simulink model "PLANTA_CONTROL_OBS"  (R2024b)
settings: Solver=FixedStepAuto  StartTime=0.0  StopTime=inf  FixedStep=0.001  MaxStep=0.0005  RelTol=1e-4
InitFcn:
  | load('ml_breakpoints.mat')
  | load('l_breakpoints.mat')
  | load('at_breakpoints.mat')
  | load('Kp_table.mat')
  | load('Kd_table.mat')
undefined symbols (not defined in the file): A_hm, A_tm, at_breakpoints, at_max, b_ha, B_hm, b_ta, B_tm, bcx, bcy, bhd, bhEb, bhm, bt, btd, btm, btw, bwu, C_hm, C_tm, D_hm, D_tm, DiscIntNeverNeededParam, dl_h_ini, dx_l_ini, dx_t_ini, dx_td_ini, dxt_max, dy_l_ini, F01_a_t_max, F01_Ts1, F02_a_h_max, F02_Ts1, F03_a_h_max, F03_a_t_max, F03_dxt_max, F03_Ts1, Fhw_min, g, Hc, ih, it, Jhd_hEb, Jhm_hb, Jtd, Jtm_tb, K_hsa, K_hsia, K_tsa, K_tsia, Kcy, Kd_table, Ke_tita, Ke_w, kp_pos, Kp_table, kp_w, Ktw, kwu, l_breakpoints ... (+26)
libraries: simulink x7, spsEdgeDetectorLib x5, simulink_extras x2, dspsigops x2, vrlib x1, dspstat3 x1
(part 4 of 4)

== stateflow chart PLANTA_CONTROL_OBS/Nivel 1 - Control Supervisor ==
  state PERFIL_DE_OBSTACULOS [parallel]
    entry:
    num_index = floor(80/Wc);
    Y_perfil = zeros(1,num_index,'double');
    during:
    %xtd = theta_mt*pulsos_x_rev*dist_x_pulso*(1/100);
    xtd_lidar = (xtd+30)+3;
    index = floor(xtd_lidar/Wc);
    Y_c0_read = yc0_xt;
    if index>0 && index<=32
    Y_perfil(index) = Y_c0_read;
    end
    settings: executionOrder=2
  state OFF [parallel]
    settings: executionOrder=1
    state EMERGENCIA
      entry:
      %Cuando el control supervisor entra en esta de emergencia, cede
      %el control al Nivel 0 hasta retomar el estado normal
      dxt_ref=0;
      dlh_ref=0;
      ddxt_ref=0;
    state ON
      entry:
      dxt_ref_ant = 0;
      dlh_ref_ant = 0;
      dxt_ref = 0;
      dlh_ref = 0;
      ddxt_ref = 0;
      state DETECCION_ESTADOS [parallel]
        settings: executionOrder=1
        state TWISTLOCKS [parallel]
          settings: executionOrder=1
          state VERIFICAR
          state ACT_TLK
            entry:
            TLK=1;
            c=-ceil((xtd+30)/Wc);
            during:
            y_real=45-(lh+Hc);
          state DES_TLK
            entry:
            TLK=0;
            c=ceil((xtd+30)/Wc);
            during:
            y_real=45-lh;
          (default) -> VERIFICAR
          VERIFICAR -> ACT_TLK [order 2] : [TLK_act==1]
          VERIFICAR -> DES_TLK [order 1] : [TLK_act==0]
          ACT_TLK -> DES_TLK : [TLK_act==0 && op_mode==1 && cable_tenso==0]
          DES_TLK -> ACT_TLK : [TLK_act==1 && op_mode==1 && cable_tenso==0]
        state FRENOS [parallel]
          settings: executionOrder=2
          state FRENO_IZAJE [parallel]
            settings: executionOrder=1
            state FRENO_IZAJE_OFF
              entry:
              BRK_h=1;
              parar_izaje=0;
            state FRENO_IZAJE_ON
              entry:
              BRK_h=0;
              parar_izaje=1;
            (default) -> FRENO_IZAJE_ON
            FRENO_IZAJE_OFF -> FRENO_IZAJE_ON : [(abs(whm)<=whm_min && (abs(whm) < abs(whm_ant)-(whm_min*0.01)))]
            FRENO_IZAJE_ON -> FRENO_IZAJE_OFF : [abs(Thm_disp) && (abs(dlh_ref)>0.1 || dlh_ref_man~=0) && after(0.2,sec)]
          state FRENO_CARRO [parallel]
            settings: executionOrder=2
            state FRENO_CARRO_OFF
              entry:
              BRK_t=1;
              parar_carro=0;
            state FRENO_CARRO_ON
              entry:
              BRK_t=0;
              parar_carro=1;
            (default) -> FRENO_CARRO_ON
            FRENO_CARRO_OFF -> FRENO_CARRO_ON : [(abs(wtm)<=wtm_min && (abs(wtm)<abs(wtm_ant)-wtm_min*0.01))]
            FRENO_CARRO_ON -> FRENO_CARRO_OFF : [abs(Ttm_disp) && (abs(dxt_ref)>0.1 || dxt_ref_man~=0) && after(0.2,sec)]
        state FINALES [parallel]
          settings: executionOrder=3
          state FIN_CARRERA_CARRO [parallel]
            settings: executionOrder=1
            state PARAR_CARRO
              entry:
              op_mode=1;
              parar_carro=1;
            state MOVER_CARRO
              entry:
              parar_carro=0;
            (default) -> MOVER_CARRO
            OFF.ON.DETECCION_ESTADOS.FINALES.FIN_CARRERA_CARRO.PARAR_CARRO -> MOVER_CARRO : [xt_ref<0 && dxt_ref>0 || xt_ref>0 && dxt_ref<0]
            MOVER_CARRO -> OFF.ON.DETECCION_ESTADOS.FINALES.FIN_CARRERA_CARRO.PARAR_CARRO : [(FC_DER==1 && dxt_ref>0) || (FC_IZQ==1 && dxt_ref<0)]
          state FIN_CARRERA_IZAJE [parallel]
            settings: executionOrder=2
            state PARAR_CARGA
              entry:
              op_mode=1;
              parar_carga=1;
            state MOVER_CARGA
              entry:
              parar_carga=0;
            (default) -> MOVER_CARGA
            PARAR_CARGA -> MOVER_CARGA : [whm<=0.3]
            MOVER_CARGA -> PARAR_CARGA : [(FC_SUP==1 && dlh_ref>0) || (FC_INF && dlh_ref<0)]
        state CONTROL_BALANCEO [parallel]
          settings: executionOrder=4
          state BALANCEO_ON
            entry:
            bal_control=1;
          state BALANCEO_OFF
            entry:
            bal_control=0;
          (default) -> BALANCEO_ON
          BALANCEO_ON -> BALANCEO_OFF : [~balanceo_on || falla_E~=0]
          BALANCEO_OFF -> BALANCEO_ON : [balanceo_on]
        state TENSION_CABLE_IZAJE [parallel]
          settings: executionOrder=5
          state TENSO
            entry:
            cable_tenso=1;
          state FLOJO
            entry:
            cable_tenso=0;
          (default) -> TENSO
          TENSO -> FLOJO : [Fhw < Fhw_min]
          FLOJO -> TENSO : [Fhw >= Fhw_min]
      state SUPERVISION [parallel]
        settings: executionOrder=2
        state ENCLAVAMIENTO_MASA [parallel]
          settings: executionOrder=3
          state INICIO
            entry:
            Ml_estimada=15000;
            dlh_max_estimada=3;
            aceptar_carga=0;
          state ESTABILIZACION
            entry:
            contador_fuerza_estable = 0;
            fuerza_estabilizada=0;
            N_estable=50;
            Fhw_ant=Fhw;
            during:
            if(abs(Fhw-Fhw_ant)<1000)
            contador_fuerza_estable = contador_fuerza_estable + 1;
            else
            contador_fuerza_estable = 0;
            end
            if contador_fuerza_estable >= N_estable
            fuerza_estabilizada = 1;
            else
            fuerza_estabilizada = 0;
            end
            Fhw_ant = Fhw;
          state ACEPTAR_CARGA
            entry:
            Ml_estimada=Ml;
            dlh_max_estimada=dlh_max;
            aceptar_carga=1;
          (default) -> INICIO
          ACEPTAR_CARGA -> INICIO : [TLK==0]
          INICIO -> ESTABILIZACION : [TLK==1 && cable_tenso==1]
          ESTABILIZACION -> ACEPTAR_CARGA : [fuerza_estabilizada==1]
        state DETECION_SOBRECARGA [parallel]
          settings: executionOrder=1
          state NORMAL
            entry:
            sobrecarga=0;
          state SOBRECARGA
            entry:
            sobrecarga=1;
          (default) -> NORMAL
          NORMAL -> OFF.ON.SUPERVISION.DETECION_SOBRECARGA.SOBRECARGA : [cable_tenso && ((Ml_estimada-Ms) > Mc_max) && aceptar_carga==1]
          OFF.ON.SUPERVISION.DETECION_SOBRECARGA.SOBRECARGA -> NORMAL : [cable_tenso == 0]
        state CONTROL_SOBREVELOCIDAD [parallel]
          settings: executionOrder=2
          state ON
            state SP_CARRO [parallel]
              settings: executionOrder=1
              state CARRO
                during:
                dxt_sp=dxt_ref_man;
              state SOBRE_dxt_MIN
                entry:
                dxt_sp=-dxt_max;
              state SOBRE_dxt_MAX
                entry:
                dxt_sp=dxt_max;
              (default) -> OFF.ON.SUPERVISION.CONTROL_SOBREVELOCIDAD.ON.SP_CARRO.CARRO
              SOBRE_dxt_MIN -> OFF.ON.SUPERVISION.CONTROL_SOBREVELOCIDAD.ON.SP_CARRO.CARRO : [dxt_ref_man >= -dxt_max]
              OFF.ON.SUPERVISION.CONTROL_SOBREVELOCIDAD.ON.SP_CARRO.CARRO -> SOBRE_dxt_MIN [order 2] : [dxt_ref_man < -dxt_max]
              SOBRE_dxt_MAX -> OFF.ON.SUPERVISION.CONTROL_SOBREVELOCIDAD.ON.SP_CARRO.CARRO : [dxt_ref_man <= dxt_max]
              OFF.ON.SUPERVISION.CONTROL_SOBREVELOCIDAD.ON.SP_CARRO.CARRO -> SOBRE_dxt_MAX [order 1] : [dxt_ref_man > dxt_max]
            state SP_IZAJE [parallel]
              settings: executionOrder=2
              state IZAJE
                during:
                dlh_sp=dlh_ref_man;
              state SOBRE_dhl_MIN
                entry:
                dlh_sp=-dlh_max_estimada
              state SOBRE_dhl_MAX
                entry:
                dlh_sp=dlh_max_estimada
              (default) -> OFF.ON.SUPERVISION.CONTROL_SOBREVELOCIDAD.ON.SP_IZAJE.IZAJE
              SOBRE_dhl_MIN -> OFF.ON.SUPERVISION.CONTROL_SOBREVELOCIDAD.ON.SP_IZAJE.IZAJE : [dlh_ref_man >= -dlh_max_estimada]
              OFF.ON.SUPERVISION.CONTROL_SOBREVELOCIDAD.ON.SP_IZAJE.IZAJE -> SOBRE_dhl_MIN [order 2] : [dlh_ref_man < -dlh_max_estimada]
              SOBRE_dhl_MAX -> OFF.ON.SUPERVISION.CONTROL_SOBREVELOCIDAD.ON.SP_IZAJE.IZAJE : [dlh_ref_man <= dlh_max_estimada]
              OFF.ON.SUPERVISION.CONTROL_SOBREVELOCIDAD.ON.SP_IZAJE.IZAJE -> SOBRE_dhl_MAX [order 1] : [dlh_ref_man > dlh_max_estimada]
          (default) -> OFF.ON.SUPERVISION.CONTROL_SOBREVELOCIDAD.ON
      state OPERACION [parallel]
        entry:
        xt_ref = xtd;
        lh_ref = 20;
        settings: executionOrder=3
        state MODO_MANUAL
          entry:
          op_mode=1;
          state CARRO [parallel]
            settings: executionOrder=1
            state CARRO_ON
              during:
              [xt_ref, dxt_ref, ddxt_ref]=limitar_aceleracion_x(dxt_sp,xtd);
            state DIST_FDC_IZQ
              during:
              [xt_ref, dxt_ref, ddxt_ref]=limitar_aceleracion_x(dxt_sp*(30+xtd)/11,xtd);
            state PARAR_CARRO
              entry:
              dxt_ref=0;
            state DIST_FDC_DER
              during:
              [xt_ref, dxt_ref, ddxt_ref]=limitar_aceleracion_x(dxt_sp*(50-xtd)/11,xtd);
            state SOBRECARGA
              entry:
              dxt_ref=0;
            (default) -> CARRO_ON
            CARRO_ON -> DIST_FDC_IZQ [order 1] : [xtd <= -19  && dxt_sp < 0 && parar_carro == 0]
            CARRO_ON -> OFF.ON.OPERACION.MODO_MANUAL.CARRO.PARAR_CARRO [order 4] : [parar_carro]
            DIST_FDC_IZQ -> CARRO_ON : [(xtd > -19 && dxt_sp > 0) || parar_carro == 1 ]
            OFF.ON.OPERACION.MODO_MANUAL.CARRO.PARAR_CARRO -> CARRO_ON : [~parar_carro]
            CARRO_ON -> DIST_FDC_DER [order 2] : [xtd >= 39  && dxt_sp > 0 && parar_carro == 0]
            CARRO_ON -> OFF.ON.OPERACION.MODO_MANUAL.CARRO.SOBRECARGA [order 3] : [sobrecarga]
            OFF.ON.OPERACION.MODO_MANUAL.CARRO.SOBRECARGA -> CARRO_ON : [~sobrecarga]
            DIST_FDC_DER -> CARRO_ON : [(xtd < 39 && dxt_sp < 0) || parar_carro == 1 ]
          state IZAJE [parallel]
            settings: executionOrder=2
            state DIST_FDC_SUP
              during:
              dlh_ref=limitar_aceleracion_y(dlh_sp*(lh-5)/7,0);
            state IZAJE_ON
              during:
              dlh_ref=limitar_aceleracion_y(dlh_sp,0);
            state PARAR_IZAJE
              entry:
              dlh_ref=0;
            state DIST_FDC_INF
              during:
              dlh_ref=limitar_aceleracion_y(dlh_sp*(65-lh)/10,0);
            state SOBRECARGA
              during:
              if (dlh_sp>=0)
              dlh_ref=dlh_sp*0.1;
              else
              end
            state ALTURA_BAJA
              during:
              %Nos elevamos a aceleracion despreciable
              dlh_ref=limitar_aceleracion_y(dlh_ref_man,0)*0.08;
              exit:
              limitar_aceleracion_y(dlh_ref,1);
            (default) -> IZAJE_ON
            IZAJE_ON -> DIST_FDC_SUP [order 1] : [lh <= 12 && dlh_sp < 0 && parar_izaje == 0]
            DIST_FDC_SUP -> IZAJE_ON : [(lh > 12 && dlh_sp > 0) || parar_izaje == 1 ]
            PARAR_IZAJE -> IZAJE_ON : [~parar_izaje]
            IZAJE_ON -> DIST_FDC_INF [order 2] : [lh >= 55 && dlh_sp > 0 && parar_izaje == 0]
            IZAJE_ON -> PARAR_IZAJE [order 3] : [parar_izaje]
            DIST_FDC_INF -> IZAJE_ON : [(lh < 55 && dlh_sp > 0) && parar_izaje == 1]
            OFF.ON.OPERACION.MODO_MANUAL.IZAJE.SOBRECARGA -> IZAJE_ON : [~sobrecarga]
            IZAJE_ON -> ALTURA_BAJA [order 5] : [TLK==1 && cable_tenso==1 && aceptar_carga == 0]
            IZAJE_ON -> OFF.ON.OPERACION.MODO_MANUAL.IZAJE.SOBRECARGA [order 4] : [sobrecarga]
            ALTURA_BAJA -> IZAJE_ON : [aceptar_carga == 1]
        state MODO_AUTOMATICO
          entry:
          % 1. Configuración Inicial
          op_mode = 0; % Modo Automático
          it = 1;      % Índice de tiempo (iterador)
          % 2. Definir parámetros para la función
          % Asegúrate de que v_max, etc., sean variables conocidas en el workspace o Data Store
          x_inicial = xtd;        % Posición actual real (no la deseada anterior)
          x_final = destino;
          y_inicial = y_real;
          % 3. Generar la trayectoria COMPLETA una sola vez al entrar
          % La función devuelve una matriz 'consignas' de tamaño 2 x N
          % Fila 1: Referencia X, Fila 2: Referencia lh
          trayectoria = gen_coords(Y_c0, dlh_max_estimada, xtd, destino,y_real);
          % Obtener la longitud de la maniobra
          dims = size(trayectoria);
          % Capturar el tiempo exacto de inicio de la maniobra
          % 't_sim' debe ser una entrada al chart proveniente del bloque 'Clock' de Simulink
          it_ultimo=0;
          dims = size(trayectoria);
          it_max = dims(2);
          during:
          % Asignación de referencias (Igual que antes)
          if(it<it_max)
          xt_ref  = trayectoria(1, it);
          lh_ref  = trayectoria(2, it);
          dxt_ref = trayectoria(3, it);
          dlh_ref = trayectoria(4, it);
          ddxt_ref = trayectoria(5, it);
          end
          it=it+1;
          exit: % Condición de salida (Fin de trayectoria)
          dxt_ref_ant = dxt_ref;
          dlh_ref_ant = dlh_ref;
          ddxt_ref_ant = ddxt_ref;
        (default) -> MODO_MANUAL
        MODO_AUTOMATICO -> MODO_MANUAL [order 2] : [dxt_ref_man ~= 0 || dlh_ref_man ~= 0]
        MODO_AUTOMATICO -> MODO_MANUAL [order 3] : [((y_real < (yc0_xt+4)) && abs(tita_l)<=tita_l_max_estable) && abs(wtm)<=wtm_min ]
        MODO_MANUAL -> MODO_AUTOMATICO : [(y_real >= (yc0_xt+4)) && (dxt_ref_man == 0 && dlh_ref_man == 0) && (~parar_carro) && after(1,sec) ]
        MODO_AUTOMATICO -> MODO_MANUAL [order 1] : [FC_DER || FC_IZQ || FC_SUP || FC_INF]
      state VIVO [parallel]
        settings: executionOrder=4
        state WAIT
          entry:
          alive=0;
        state TALK
          entry:
          alive=1;
        (default) -> WAIT
        WAIT -> TALK : [after(500,msec)]
        TALK -> WAIT : [after(20,msec)]
    (default) -> OFF.ON
    EMERGENCIA -> OFF.ON : [~falla_E]
    OFF.ON -> EMERGENCIA : [falla_E]
  data: xt_manual function_output; dx_manual function_input; vel_maxima_x function_output; F01_a_t_max parameter; F01_Ts1 parameter; a_maxima_x function_output; x_actual function_input; dy_manual function_input; v_maxima_y function_output; estado function_input; at_max parameter; F02_Ts1 parameter; F02_a_h_max parameter; perfil_modif function_input; v_max_izaje function_input; x_inicio function_input; x_destino function_input; y_inicio function_input; F03_Ts1 parameter; consignas function_output; F03_dxt_max parameter; F03_a_t_max parameter; xx_c0 parameter; F03_a_h_max parameter; dxt_ref output; dlh_ref output; Mc_max parameter double; y_inicial local double size=1; Fhw input; Fhw_min parameter; Ml input; FC_SUP input; FC_INF input; FC_IZQ input; FC_DER input; xtd input; x_inicial local size=1; x_fin_consigna local =0; pos_ref local size=[2 400000]; parametros local; num_index local; it_fin local =20000; it local; index local; cable_tenso local double; Y_c0_read local; TLK output =0; Kp local; xtd_lidar local; c output =2000; bal_control output size=1; Y_perfil local double size=[1, floor(80/Wc)]; whm input; whm_ant input; wtm input; wtm_ant input; whm_min parameter; wtm_min parameter; lh input; falla_E input; dlh_max input; dlh_ref_man input; dxt_ref_man input; BRK_h output; BRK_t output; destino input; balanceo_on input; TLK_act input; Wc parameter; T_s1 parameter; parar_izaje local double; parar_carro local double; parar_carga local; alive output double =1; emergency local; dxt_max parameter; dxt_sp local =0; dlh_sp local =0; tol_lh local; tol_x local; lh_max_permitida local; i local; Y_c0 input; yc0_xt input; dims local; trayectoria local size=[5 400000]; x_final local; it_max local; v_h_max local; it_calculado local; t_inicio local; pausa_global local; it_ultimo local; dtsimu local; Hc parameter; y_real local =0; dxt_ref_ant local; dlh_ref_ant local; Ttm_disp input =1; Thm_disp input =1; rhd parameter; ih parameter; aceptar_carga local double; fuerza_estabilizada local; contador_fuerza_estable local; N_estable local; Fhw_ant local; Ms parameter; Ml_estimada output =0; ddxt_ref output; xt_ref output; lh_ref output; ddxt_ref_ant local; tita_l input; tita_l_max_estable parameter; BRK_hE local; dlh_max_estimada output; sobrecarga output double =0; op_mode output double; dxt_ref_prev local
  function [xt_manual, vel_maxima_x, a_maxima_x] = limitar_aceleracion_x(dx_manual,x_actual):
    | function [xt_manual, vel_maxima_x, a_maxima_x] = limitar_aceleracion_x(dx_manual,x_actual)
    | 
    | persistent dx_tref_manual_ant
    | persistent dx_tref_manual_ant_2
    | 
    | %x0 = xt_ref;
    | 
    | %Asignacion de variables externas
    | a_t_max=F01_a_t_max;
    | tiempo_muestreo=F01_Ts1;
    | 
    | if isempty(dx_tref_manual_ant)
    |     dx_tref_manual_ant=0;
    | end
    | if isempty(dx_tref_manual_ant_2)
    |     dx_tref_manual_ant_2=0;
    | end
    | if abs(dx_manual)>=abs(dx_tref_manual_ant)
    |     if dx_manual>0
    |         v_max=a_t_max*tiempo_muestreo+dx_tref_manual_ant;
    |         if dx_manual>v_max
    |              vel_maxima_x=v_max;
    |         else 
    |             vel_maxima_x=dx_manual;
    |         end
    | 
    |     else 
    |         v_max=-a_t_max*tiempo_muestreo+dx_tref_manual_ant;
    |         if dx_manual<v_max
    |             vel_maxima_x=v_max;
    |         else 
    |             vel_maxima_x=dx_manual;
    |         end
    |     end
    | else
    |     if dx_manual<dx_tref_manual_ant
    |         v_max=-a_t_max*tiempo_muestreo+dx_tref_manual_ant;
    |         if dx_manual<v_max
    |              vel_maxima_x=v_max;
    |         else 
    |             vel_maxima_x=dx_manual;
    |         end
    | 
    |     else 
    |         v_max=a_t_max*tiempo_muestreo+dx_tref_manual_ant;
    |         if dx_manual>v_max
    |             vel_maxima_x=v_max;
    |         else 
    |             vel_maxima_x=dx_manual;
    |         end
    |     end
    | end
    | a_maxima_x = (vel_maxima_x-dx_tref_manual_ant_2)/2*tiempo_muestreo;
    | %xt_manual = x0+(dx_tref_manual_ant_2+4*dx_tref_manual_ant+vel_maxima_x)*tiempo_muestreo/3;
    | xt_manual = x_actual;
    | dx_tref_manual_ant_2=dx_tref_manual_ant;
    | dx_tref_manual_ant=vel_maxima_x;
    | end
  function v_maxima_y = limitar_aceleracion_y(dy_manual,estado):
    | function v_maxima_y = limitar_aceleracion_y(dy_manual,estado)
    | 
    | persistent dy_href_manual_ant
    | 
    | % Asignacion de variables externas
    | a_h_max = F02_a_h_max;
    | tiempo_muestreo = F02_Ts1;
    | 
    | if isempty(dy_href_manual_ant)
    |     dy_href_manual_ant = 0;
    | end
    | 
    | if estado == 0
    | 
    |     % Detectar cambio de signo
    |     if dy_manual * dy_href_manual_ant < 0
    |         dy_href_manual_ant = 0;
    |     end
    | 
    |     delta = dy_manual - dy_href_manual_ant;
    |     delta_max = a_h_max * tiempo_muestreo;
    | 
    |     if delta > delta_max
    |         delta = delta_max;
    |     elseif delta < -delta_max
    |         delta = -delta_max;
    |     end
    | 
    |     v_maxima_y = dy_href_manual_ant + delta;
    | 
    |     dy_href_manual_ant = v_maxima_y;
    | 
    | else
    | 
    |     v_maxima_y = dy_manual;
    |     dy_href_manual_ant = dy_manual;
    | 
    | end
    | 
    | end
    | % function v_maxima_y = limitar_aceleracion_y(dy_manual,estado)
    | % 
    | % persistent dy_href_manual_ant
    | % 
    | % Asignacion de variables externas
    | % a_h_max=F02_a_h_max;
    | % tiempo_muestreo=F02_Ts1;
    | % 
    | % if isempty(dy_href_manual_ant)
    | %     dy_href_manual_ant=0;
    | % end
    | % if estado==0
    | %     if abs(dy_manual)>=abs(dy_href_manual_ant)
    | %         if dy_manual>0
    | %             v_max=a_h_max*tiempo_muestreo+dy_href_manual_ant;
    | %             if dy_manual>v_max
    | %                 v_maxima_y=v_max;
    | %             else 
    | %                 v_maxima_y=dy_manual;
    | %             end
    | % 
    | %         else 
    | %             v_max=-a_h_max*tiempo_muestreo+dy_href_manual_ant;
    | %             if dy_manual<v_max
    | %                 v_maxima_y=v_max;
    | %             else 
    | %                 v_maxima_y=dy_manual;
    | %             end
    | %         end
    | %     else
    | %         if dy_manual<dy_href_manual_ant
    | %             v_max=-a_h_max*tiempo_muestreo+dy_href_manual_ant;
    | %             if dy_manual<v_max
    | %                  v_maxima_y=v_max;
    | %             else 
    | %                 v_maxima_y=dy_manual;
    | %             end
    | % 
    | %         else 
    | %             v_max=a_h_max*tiempo_muestreo+dy_href_manual_ant;
    | %             if dy_manual>v_max
    | %                 v_maxima_y=v_max;
    | %             else 
    | %                 v_maxima_y=dy_manual;
    | %             end
    | %         end
    | %     end
    | %     dy_href_manual_ant=v_maxima_y;
    | % else 
    | %     dy_href_manual_ant=dy_manual;
    | % end
    | % end
  function consignas = gen_coords(perfil_modif,v_max_izaje,x_inicio,x_destino,y_inicio):
    | function consignas = gen_coords(perfil_modif,v_max_izaje,x_inicio,x_destino,y_inicio)
    | %consignas: Matriz 2xn con referencias en x y lh muestreadas
    | %Y_c0_vector_modif: Perfil de obstaculos (altura)
    | %v_max_izaje_valor: Vel maxima de izaje (en eje vertical)
    | %x_t_inicial, x_t_final: Posicion inicial y final en X
    | %y_l_inicial: Altura inicial (y, no lh)
    | %sample_time: periodo de muestreo
    | 
    | %% Inicio Funcion
    | %Asignación de variables externas
    | ah_max=F03_a_h_max; %Aceleracion max de izaje
    | at_max=F03_a_t_max; %Aceleracion max de carro
    | vt_max=F03_dxt_max; %Velocidad max carro
    | Ts=0.02; %Muestreo sistema de control N1
    | 
    | % Parámetros locales
    | x_ini = x_inicio
    | x_fin = x_destino
    | y_ini = y_inicio    % altura inicial (y)
    | vh_max = v_max_izaje;
    | margen_seg = 3;        
    | perfil_seg = perfil_modif+margen_seg;
    | 
    | % Índices del perfil y límites de seguridad
    | idx_ini = round((x_ini+30)/2.44);
    | idx_fin = round((x_fin+30)/2.44);
    | idx_ini = max(1, min(idx_ini, length(perfil_seg)));
    | length(idx_ini)
    | idx_fin   = max(1, min(idx_fin, length(perfil_seg)));
    | length(idx_fin)
    | y_fin = perfil_seg(idx_fin);
    | 
    | %% Obtenemos el perfil de obstáculos en el tramo
    | 
    | % Determinamos lo indices i_min e i_max de menor a mayor
    | i_min = min(idx_ini, idx_fin);
    | i_max = max(idx_ini, idx_fin);
    | 
    | % Extraemos el perfil seguro y perfil de obstaculos siempre de menor a
    | % mayor para evitar que se asigne vacio
    | perfil = perfil_seg;
    | perfil_rec = perfil_seg(i_min:i_max);
    | 
    | %Si el movimiento de izquierda a derecha, se mantiene la asignacion
    | 
    | %Si el movimiento es de derecha a izquierda, se invierte el recorrido de
    | %los vectores
    | if idx_ini > idx_fin
    |     perfil = flip(perfil)
    |     perfil_rec = flip(perfil_rec)
    | end
    | 
    | % %% Trayecto 1: Primer parte de la trayectoria
    | % %Revisamos alrededores para evitar colisiones
    | % if (y_inicio <= perfil(idx_ini+1*sign(idx_fin-idx_ini)))
    | %     y_ini_1 = y_ini
    | %     y_fin_1 = perfil(idx_ini+1*sign(idx_fin-idx_ini))
    | %     x_ini_1 = x_ini
    | %     x_fin_1 = x_ini
    | %     t_v_y_1 = (abs(y_fin_1-y_ini_1)/vh_max)+vh_max/ah_max;
    | % 
    | % else
    | %     y_ini_1 = y_ini
    | %     y_fin_1 = y_ini
    | % 
    | %     t_v_y_1 = 0.1
    | %     x_ini_1 = x_ini
    | %     x_fin_1 = x_ini
    | % end
    | 
    | %% Trayecto 2: Parabola/Arco Ascendente
    | y_ini_2 = y_ini
    | x_ini_2 = x_ini
    | 
    | % Buscamos altura maxima de obstaculo
    | [y_max_obs, idx_max_obs] = max(perfil_rec)
    | y_fin_2 = y_max_obs+1
    | x_fin_2 = 2.44*(idx_ini+idx_max_obs*sign(idx_fin-idx_ini))-30 % -----------------------JUANI---------------------------------
    | 
    | t_v_y_2 = (abs(y_fin_2-y_ini_2)/vh_max)+vh_max/ah_max;
    | t_v_x_2 = (abs(x_fin_2-x_ini_2)/vt_max)+vt_max/at_max;
    | 
    | 
    | 
    | %% Trayecto 3: Parabola/Arco Descendente
    | y_ini_3 = y_fin_2
    | x_ini_3 = x_fin_2
    | x_fin_3 = x_fin
    | 
    | % Revisamos los alrededores del final para evitar colisiones
    | if (y_fin <= perfil(idx_fin+1*sign(idx_fin-idx_ini)))
    |     y_fin_3 = perfil(idx_fin+1*sign(idx_fin-idx_ini))
    | else
    |     y_fin_3 = y_fin
    | end
    | 
    | t_v_y_3 = t_v_y_2+(abs(y_fin_3-y_ini_3)/vh_max)+vh_max/ah_max;
    | t_v_x_3 = t_v_x_2+(abs(x_fin_3-x_ini_3)/vt_max)+vt_max/at_max;
    | 
    | 
    | 
    | 
    | 
    | t_hitos_y = [0, t_v_y_2, t_v_y_3]
    | length(t_hitos_y);
    | t_hitos_x = [0, t_v_x_2, t_v_x_3]
    | length(t_hitos_x);
    | x_hitos = [x_ini, x_fin_2, x_fin_3]
    | length(x_hitos);
    | y_hitos = [y_ini, y_fin_2, y_fin_3]
    | length(y_hitos);
    | t_v_max = max(t_v_y_3,t_v_x_3)
    | t_vec_new = 0:Ts:t_v_max;
    | length(t_vec_new)
    | 
    | x_ref = spline(t_hitos_x, [0, x_hitos, 0], t_vec_new);
    | y_ref = spline(t_hitos_x, [0,y_hitos, 0], t_vec_new);
    | 
    | %Convertimos la referencia a lh
    | y_ref=45-y_ref;
    | 
    | 
    | consignas = zeros(5,length(t_vec_new));
    | 
    | 
    | vx_ref = gradient(x_ref,Ts);
    | vy_ref = gradient(y_ref,Ts);
    | ax_ref = gradient(vx_ref,Ts);
    | 
    | 
    | 
    | consignas(1,:) = x_ref;
    | consignas(2,:) = 45-y_ref;
    | consignas(3,:) = vx_ref;
    | consignas(4,:) = vy_ref;
    | consignas(5,:) = ax_ref;
    | 
    | end

== stateflow chart PLANTA_CONTROL_OBS/Nivel 0 - Seguridad o Proteccion ==
  settings: updateMethod=DISCRETE  sampleTime=T_s0
  state CONTROL_SEGURIDAD
    state Verificacion
      entry:
      EmergenciaNivel = 0;
      BRK_t = 1;
      BRK_h = 1;
      BRK_hE = 1;
      cont=0;
      state VERIFICA_WATCHDOG [parallel]
        entry:
        cont = 0;
        settings: executionOrder=1
        state ALIVE
          entry:
          cont = 0;
        state WAIT
        state EMERGENCIA_N1
          entry:
          EmergenciaNivel = 1;
        state CONTADOR
          entry:
          cont = cont + 1;
        (default) -> CONTROL_SEGURIDAD.Verificacion.VERIFICA_WATCHDOG.WAIT
        CONTROL_SEGURIDAD.Verificacion.VERIFICA_WATCHDOG.WAIT -> ALIVE [order 3] : [hasChanged(alive)]
        CONTROL_SEGURIDAD.Verificacion.VERIFICA_WATCHDOG.WAIT -> CONTROL_SEGURIDAD.Verificacion.VERIFICA_WATCHDOG.EMERGENCIA_N1 [order 1] : [cont >= 5]
        ALIVE -> CONTROL_SEGURIDAD.Verificacion.VERIFICA_WATCHDOG.WAIT : [true]
        CONTADOR -> CONTROL_SEGURIDAD.Verificacion.VERIFICA_WATCHDOG.WAIT : [true]
        CONTROL_SEGURIDAD.Verificacion.VERIFICA_WATCHDOG.WAIT -> CONTADOR [order 2] : after(1,sec)
      state VERIFICA_FIN_CARRERA [parallel]
        settings: executionOrder=3
        state EMERGENCIA_N2
          entry:
          EmergenciaNivel = 2;
        state WAIT
        state EMERGENCIA_N3
          entry:
          EmergenciaNivel = 3;
        CONTROL_SEGURIDAD.Verificacion.VERIFICA_FIN_CARRERA.WAIT -> CONTROL_SEGURIDAD.Verificacion.VERIFICA_FIN_CARRERA.EMERGENCIA_N2 [order 1] : [FCE_SUP || FCE_INF]
        (default) -> CONTROL_SEGURIDAD.Verificacion.VERIFICA_FIN_CARRERA.WAIT
        CONTROL_SEGURIDAD.Verificacion.VERIFICA_FIN_CARRERA.WAIT -> EMERGENCIA_N3 [order 2] : [FCE_DER || FCE_IZQ]
      state VERIFICA_PULSADOR [parallel]
        settings: executionOrder=2
        state WAIT
        state EMERGENCIA_N1
          entry:
          EmergenciaNivel = 1;
        (default) -> CONTROL_SEGURIDAD.Verificacion.VERIFICA_PULSADOR.WAIT
        CONTROL_SEGURIDAD.Verificacion.VERIFICA_PULSADOR.WAIT -> CONTROL_SEGURIDAD.Verificacion.VERIFICA_PULSADOR.EMERGENCIA_N1 : [PulsadorEmergecia == 1]
      state VERIFICA_SOBREVELOCIDAD [parallel]
        settings: executionOrder=4
        state WAIT
        state EMERGENCIA_N2
          entry:
          EmergenciaNivel = 2;
        (default) -> CONTROL_SEGURIDAD.Verificacion.VERIFICA_SOBREVELOCIDAD.WAIT
        CONTROL_SEGURIDAD.Verificacion.VERIFICA_SOBREVELOCIDAD.WAIT -> CONTROL_SEGURIDAD.Verificacion.VERIFICA_SOBREVELOCIDAD.EMERGENCIA_N2 : [ dlh>= 1.15*v_max_izaje]
    state Emergencia_TOTAL
      entry:
      BRK_t = 0;
      BRK_h = 0;
      BRK_hE = 0;
    state Emergencia_IZAJE
      entry:
      BRK_h = 0;
      BRK_hE = 0;
    state Emergencia_CARRO
      entry:
      BRK_t = 0;
    (default) -> Verificacion
    Emergencia_TOTAL -> Verificacion : [OK]
    Verificacion -> Emergencia_TOTAL [order 1] : [EmergenciaNivel == 1]
    Emergencia_IZAJE -> Verificacion : [OK]
    Verificacion -> Emergencia_IZAJE [order 2] : [EmergenciaNivel == 2]
    Emergencia_CARRO -> Verificacion : [OK]
    Verificacion -> Emergencia_CARRO [order 3] : [EmergenciaNivel == 3]
  data: alive input; BRK_h output; BRK_t output; FCE_DER input; FCE_IZQ input; FCE_INF input; FCE_SUP input; PulsadorEmergecia input; cont local; v_max_izaje input; dlh input; EmergenciaNivel output =0; OK input; BRK_hE output

== matlab function PLANTA_CONTROL_OBS/sensor ==
  data: y0_array input; distancia output; index input; Yt0 parameter
function distancia= mideDistancia(y0_array,index, Yt0)


if (index>0 && index<=32)
    distancia = Yt0-y0_array(index);
else
   distancia = Yt0;
end

== stateflow chart PLANTA_CONTROL_OBS/Enclavamiento ==
  state Espera
  state Cambiar
    entry:
    output=(~output);
  (default) -> Espera
  Espera -> Cambiar : [input]
  Cambiar -> Espera : [input==0]
  data: input input; output output boolean =false

== matlab function PLANTA_CONTROL_OBS/Calculo ==
  data: masas_array input; Mc_X output; index input
function Mc_X= calcula_Mc_X(masas_array,index)
if (index>0 && index<=32)
    Mc_X =masas_array(index);
else
    Mc_X=0;
end

== stateflow chart PLANTA_CONTROL_OBS/Enclavamiento1 ==
  state Espera
  state Cambiar
    entry:
    output=(~output);
  (default) -> Espera
  Espera -> Cambiar : [input]
  Cambiar -> Espera : [input==0]
  data: input input; output output boolean =false

== matlab function PLANTA_CONTROL_OBS/Velocidad max izaje ==
  data: M_l input; dxt_max output
function dxt_max = fcn(M_l)

Pnom=956.15e3; %Potencia nominal motor
g= 9.80665; %Acel gravitatoria

if (M_l>=65000)
    dxt_max = 1.5; %1.5 m/s
elseif (32500<=M_l)&&(M_l<65000)
    dxt_max = Pnom/(M_l*g);
elseif (M_l<32500)
    dxt_max=3; %3 m/s
else
    dxt_max = 1.5;

end

== matlab function PLANTA_CONTROL_OBS/PLANTA/Masa de contenedor (A partir de posicion x_l)/Calculo ==
  data: masas_array input; Mc_X output; index input
function Mc_X= calcula_Mc_X(masas_array,index)

if (index>0 && index<=32)
    Mc_X =masas_array(index);
else
    Mc_X=0;

end

== matlab function PLANTA_CONTROL_OBS/Actualizar perfil/Enabled Subsystem/Actualiza perfil ==
  data: index input; y0_actualizado output; y0 input; Hc input
function y0_actualizado = fcn(index,y0,Hc)
y0_anterior=y0;
if (abs(index)>0 && abs(index)<=32)
y0_anterior(abs(index))=y0_anterior(abs(index))+Hc*sign(index);
y0_actualizado=y0_anterior;
else
y0_actualizado=y0;
end
